simulink model "Problem8"  (R2020b)
settings: Solver=VariableStepAuto  StartTime=0.0  StopTime=inf  RelTol=1e-3
settings Model: Creator=HP  LastModifiedBy=HP

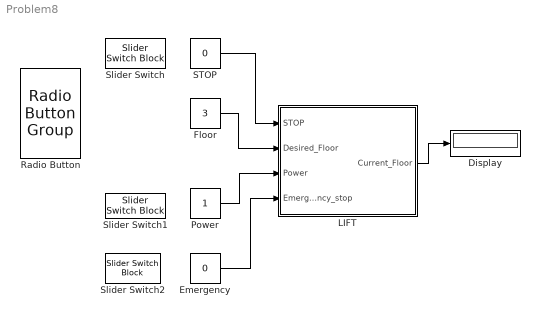
== system Problem8 ==
  Display : Display
  Emergency : Constant  Value=0
  Floor : Constant  Value=3
  "LIFT " : Stateflow chart  TreatAsAtomicUnit=on
  Power : Constant
  Radio Button : RadioButtonGroup  LabelPosition=Bottom  SelectedLabel=Third Floor  ButtonGroupName=Group
      settings: Values={{'First  Floor', 'Second Floor', 'Third Floor', 'Fourth Floor', 'Fifth Floor'}, [1 2 3 4 5]}
  STOP : Constant  Value=0
  Slider Switch : SliderSwitchBlock
      settings: Values={{'Off', 'On'}, [0 1]}
  Slider Switch1 : SliderSwitchBlock
      settings: Values={{'Off', 'On'}, [0 1]}
  Slider Switch2 : SliderSwitchBlock
      settings: Values={{'Off', 'On'}, [0 1]}
  wires:
  STOP/1 -> "LIFT "/1(STOP)
  "LIFT "/1(Current_Floor) -> Display/1
  Floor/1 -> "LIFT "/2(Desired_Floor)
  Power/1 -> "LIFT "/3(Power)
  Emergency/1 -> "LIFT "/4(Emergency_stop)

== stateflow chart Problem8/LIFT  ==
  state Lift [parallel]
    settings: executionOrder=1
    (history)
    state Power
    state NORMAL
      state Loop1 [parallel]
        settings: executionOrder=1
        (history)
        state Emer
          en:
        state Working
          en:
          state Off
            en:
            disp 'LIFT STOPPED';
          state On
            en:
            (history)
            state First
              entry:
              i=1;
              Current_Floor=1;
              disp '1 Floor';
            state Second
              en:
              i=2;
              Current_Floor=2;
              disp '2 Floor';
            state Third
              en:
              i=3;
              Current_Floor=3;
              disp '3 Floor';
            state Fifth
              en:
              i=5;
              Current_Floor=5;
              disp '5 Floor';
            state Fourth
              en:
              i=4;
              Current_Floor=4;
              disp '4 Floor';
            (default) -> First
            Second -> Third [order 2] : [i<Desired_Floor]
            Third -> Fourth [order 1] : [i<Desired_Floor]
            Fourth -> Fifth [order 1] : [i<Desired_Floor]
            First -> Second : [i<Desired_Floor]
            Fifth -> Fourth : [i>Desired_Floor]
            Fourth -> Third [order 2] : [i>Desired_Floor]
            Second -> First [order 1] : [i>Desired_Floor]
            Third -> Second [order 2] : [i>Desired_Floor]
          (default) -> Off
          Off -> On : [STOP==0]{disp 'LIFT RUNNING';}
          On -> Off : [STOP==1]
        (default) -> Emer
        Emer -> Working : [Emergency_stop==0]{send(No_emg,Emergency)}
        Working -> Emer : [Emergency_stop==1]{send(Emg,Emergency)}
      state Emergency [parallel]
        settings: executionOrder=2
        (history)
        state Emg_off
          en:
        state Emg_On
          en:
          disp 'EMERGENCY STOP AND ALARM ARE ON';
        (default) -> Emg_off
        Emg_off -> Emg_On : Emg
        Emg_On -> Emg_off : No_emg{disp 'EMERGENCY STOP AND ALARM ARE OFF'}
    (default) -> Power
    Power -> NORMAL : [Power==1]{disp 'Power On'}
    NORMAL -> Power : [Power==0]{disp 'Power Off'}
  data: i local; STOP input; Current_Floor output; Desired_Floor input; Power input; Emergency_stop input
  events: Emg local FUNCTION_CALL_EVENT; No_emg local FUNCTION_CALL_EVENT
